simulink model "excneuronv3"  (Simulink 7.6)
settings: Solver=ode45  StartTime=0.0  StopTime=10.0  RelTol=1e-3
values from neighbouring files (symbols this model uses):
  amp = 1    [excneuroninit.m]
  h = -0.5    [excneuroninit.m]
  maxcon = 10    [excneuroninit.m]
  neurodist = 1    [excneuroninit.m]
  sigslope = 3    [excneuroninit.m]
  tau_u = 0.05    [excneuroninit.m]
undefined symbols (not defined in the file or in its folder): ut, wvec
libraries: simulink x3
settings Model: Creator=root  LastModifiedBy=root

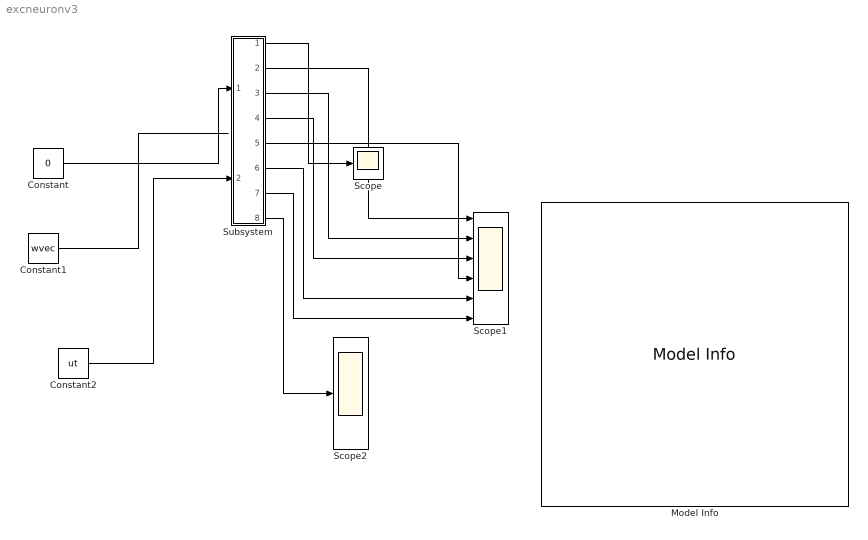
== system excneuronv3 ==
  Constant : Constant  Value=0
  Constant1 : Constant  Value=wvec
  Constant2 : Constant  Value=ut
  Model Info : simulink/Model-Wide Utilities/Model Info  SystemSampleTime=-1  InitialBlockCM=None  BlockCM=None  Frame=on  DisplayStringWithTags=|  HorizontalTextAlignment=Left  LeftAlignmentValue=0.02  SourceBlockDiagram=excneuronv3  TagMaxNumber=20
      | Excitatory neuron with support to
      |  inter population connection and intra population .
      | INPUTS
      | 1) I(t) from different neuralpools
      | 2) weight vector 
      | 3) 1st port inhibitory connection
      |  from inhibitory sub population 
      | ,remaining  2nd port to last port 
      | neurons with in excitatory sub  population
      | VARIABLES
      | 1) sigslope = sigmoid slope for non linearity in signals
      | 2)maxcon= total number of 
      | connections from intra population neurons
      | 3) amp = intra neuron weight amplitude for max neuron
      | 4)neurodist = the mean distance 
      | from the current neuron where 
      | weight is maximum (weight of intra 
      | neuron connections are based on distance between them)
      | 5) h = the threshold in leaky integrator model
      | 6) tau_u = the timeconstant for excitatory neuron
  Scope : Scope
  Scope1 : Scope  NumInputPorts=6
      settings: YMin=-5~-5~-5~-5~-5~-5  YMax=10~10~5~5~5~5
  Scope2 : Scope
      settings: YMax=10  SaveName=ScopeData2
  Subsystem : Subsystem
  wires:
  Constant/1 -> Subsystem/1(In1)
  Constant1/1 -> ?
  Constant2/1 -> Subsystem/2(In3)
  Subsystem/1(Out1) -> Scope/1
  Subsystem/2(Out2) -> Scope1/1
  Subsystem/3(Out3) -> Scope1/2
  Subsystem/4(Out4) -> Scope1/3
  Subsystem/5(Out5) -> Scope1/4
  Subsystem/6(Out6) -> Scope1/5
  Subsystem/7(Out7) -> Scope1/6
  Subsystem/8(Out8) -> Scope2/1

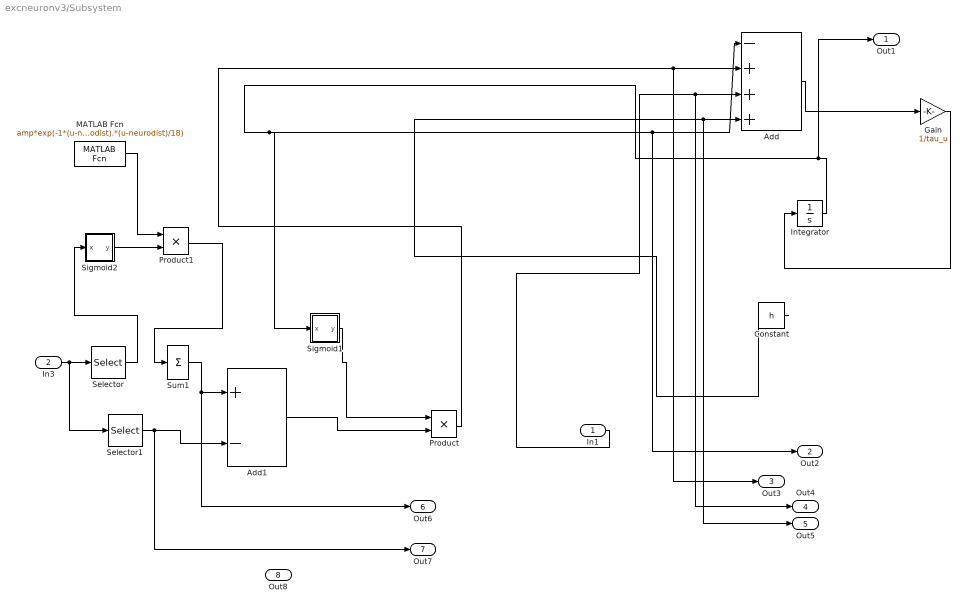
== system excneuronv3/Subsystem ==
  In1 : Inport
  In3 : Inport  Port=2
  Add : Sum  Inputs=-+++
  Add1 : Sum  Inputs=+-
  Constant : Constant  Value=h
  Gain : Gain  Gain=1/tau_u
  Integrator : Integrator  InitialCondition=1
  MATLAB Fcn : MATLABFcn  MATLABFcn=amp*exp(-1*(u-neurodist).*(u-neurodist)/18)  OutputDimensions=maxcon
  Product : Product  RndMeth=Zero
  Product1 : Product  RndMeth=Zero
  Selector : Selector  InputPortWidth=maxcon+1  IndexOptions=Starting index (dialog)  Indices=2  OutputSizes=maxcon
  Selector1 : Selector  InputPortWidth=maxcon+1  IndexOptions=Starting index (dialog)  Indices=1  OutputSizes=1
  Sigmoid1 : Subsystem  TreatAsAtomicUnit=on  mask{slope=sigslope, offset=0.5}
      mask help: Created by Han, Cheol
      mask Display: plot([10 15 20 25 30 35 40 45 50], [0 0.01 0.1 0.2 0.5 0.8 0.9 0.99 1])
  Sigmoid2 : Subsystem  TreatAsAtomicUnit=on  mask{slope=sigslope, offset=0.5}
      mask help: Created by Han, Cheol
      mask Display: plot([10 15 20 25 30 35 40 45 50], [0 0.01 0.1 0.2 0.5 0.8 0.9 0.99 1])
  Sum1 : Sum  Inputs=+  SaturateOnIntegerOverflow=on
  Out1 : Outport
  Out2 : Outport  Port=2
  Out3 : Outport  Port=3
  Out4 : Outport  Port=4
  Out5 : Outport  Port=5
  Out6 : Outport  Port=6
  Out7 : Outport  Port=7
  Out8 : Outport  Port=8
  wires:
  Add/1 -> Gain/1
  Gain/1 -> Integrator/1
  Integrator/1 -> Sigmoid1/1(x), Add/1, Out2/1, Out1/1
  Sigmoid1/1(y) -> Product/1
  Product/1 -> Add/2, Out3/1
  In1/1 -> Add/3, Out4/1
  Constant/1 -> Add/4, Out5/1
  In3/1 -> Selector/1, Selector1/1
  Product1/1 -> Sum1/1
  Selector/1 -> Sigmoid2/1(x)
  ? -> MATLAB Fcn/1
  MATLAB Fcn/1 -> Product1/1
  Sum1/1 -> Add1/1, Out6/1
  Selector1/1 -> Add1/2, Out7/1
  Sigmoid2/1(y) -> Product1/2
  Add1/1 -> Product/2

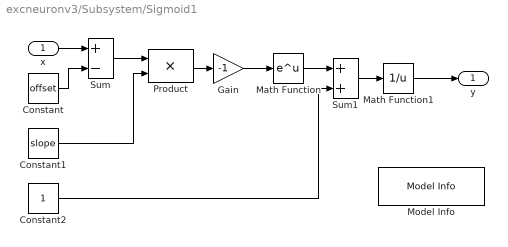
== system excneuronv3/Subsystem/Sigmoid1 ==
  x : Inport
  Constant : Constant  Value=offset
  Constant1 : Constant  Value=slope
  Constant2 : Constant
  Gain : Gain  Gain=-1  SaturateOnIntegerOverflow=on  OutDataTypeStr=Inherit: Same as input  ParamDataTypeStr=Inherit: Same as input
  Math Function : Math  SaturateOnIntegerOverflow=on
  Math Function1 : Math  Operator=reciprocal  SaturateOnIntegerOverflow=on
  Model Info : simulink/Model-Wide Utilities/Model Info  SystemSampleTime=-1  InitialBlockCM=None  BlockCM=None  Frame=on  DisplayStringWithTags=|  HorizontalTextAlignment=Center  LeftAlignmentValue=0.5  SourceBlockDiagram=excneuronv3  TagMaxNumber=20
      | Model Info
      | %<Creator> Han, Cheol
  Product : Product  SaturateOnIntegerOverflow=on  OutDataTypeStr=Inherit: Same as first input
  Sum : Sum  Inputs=+-  SaturateOnIntegerOverflow=on
  Sum1 : Sum  SaturateOnIntegerOverflow=on
  y : Outport  InitialOutput=0
  wires:
  x/1 -> Sum/1
  Constant/1 -> Sum/2
  Sum/1 -> Product/1
  Constant1/1 -> Product/2
  Product/1 -> Gain/1
  Gain/1 -> Math Function/1
  Math Function/1 -> Sum1/1
  Constant2/1 -> Sum1/2
  Sum1/1 -> Math Function1/1
  Math Function1/1 -> y/1

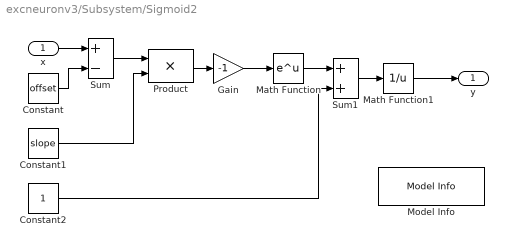
== system excneuronv3/Subsystem/Sigmoid2 ==
  x : Inport
  Constant : Constant  Value=offset
  Constant1 : Constant  Value=slope
  Constant2 : Constant
  Gain : Gain  Gain=-1  SaturateOnIntegerOverflow=on  OutDataTypeStr=Inherit: Same as input  ParamDataTypeStr=Inherit: Same as input
  Math Function : Math  SaturateOnIntegerOverflow=on
  Math Function1 : Math  Operator=reciprocal  SaturateOnIntegerOverflow=on
  Model Info : simulink/Model-Wide Utilities/Model Info  SystemSampleTime=-1  InitialBlockCM=None  BlockCM=None  Frame=on  DisplayStringWithTags=|  HorizontalTextAlignment=Center  LeftAlignmentValue=0.5  SourceBlockDiagram=excneuronv3  TagMaxNumber=20
      | Model Info
      | %<Creator> Han, Cheol
  Product : Product  SaturateOnIntegerOverflow=on  OutDataTypeStr=Inherit: Same as first input
  Sum : Sum  Inputs=+-  SaturateOnIntegerOverflow=on
  Sum1 : Sum  SaturateOnIntegerOverflow=on
  y : Outport  InitialOutput=0
  wires:
  x/1 -> Sum/1
  Constant/1 -> Sum/2
  Sum/1 -> Product/1
  Constant1/1 -> Product/2
  Product/1 -> Gain/1
  Gain/1 -> Math Function/1
  Math Function/1 -> Sum1/1
  Constant2/1 -> Sum1/2
  Sum1/1 -> Math Function1/1
  Math Function1/1 -> y/1
